simulink model "PMSM_MRAS"  (R2018b)
settings: Solver=ode23tb  StartTime=0.0  StopTime=6  FixedStep=5e-5  RelTol=1e-3  EnableMultiTasking=on
InitFcn:
  | L=8.5e-3;
  | R=2.875;
  | flux=0.175;
libraries: powerlib x5, powerlib_extras x3, simulink x1
settings Model: Creator=Paladin611  LastModifiedBy=liangjin
settings DataIOCC: SaveFormat=Array
settings OptimizationCC: ExpressionDepthLimit=2147483647  InitFltsAndDblsToZero=on  EfficientMapNaN2IntZero=off  LifeSpan=inf
settings DebuggingCC: SaveWithParameterizedLinksMsg=none  UnderspecifiedInitializationDetection=Classic  MergeDetectMultiDrivingBlocksExec=none  SignalResolutionControl=TryResolveAllWithWarning  SolverPrmCheckMsg=warning  MultiTaskDSMMsg=warning  MultiTaskCondExecSysMsg=none  FcnCallInpInsideContextMsg=warning  StateNameClashWarn=warning  SFUnexpectedBacktrackingDiag=warning  SFNoUnconditionalDefaultTransitionDiag=warning  SFExecutionAtInitializationDiag=none
settings HardwareCC: ProdBitPerPointer=32  ProdBitPerSizeT=32  ProdBitPerPtrDiffT=32  ProdLargestAtomicFloat=None  ProdIntDivRoundTo=Undefined  ProdEndianess=Unspecified  ProdWordSize=32  ProdHWDeviceType=32-bit Generic  TargetBitPerPointer=64  TargetBitPerSizeT=64  TargetBitPerPtrDiffT=64  TargetLongLongMode=on  TargetIntDivRoundTo=Zero  TargetEndianess=LittleEndian  TargetWordSize=64  TargetHWDeviceType=MATLAB Host  ProdEqTarget=off
settings ModelReferenceCC: PropagateSignalLabelsOutOfModel=off
settings SFSimCC: SimUseLocalCustomCode=off
settings RTWCC: RTWUseLocalCustomCode=off
settings CodeAppCC: MaxIdLength=128  StateflowObjectComments=on
settings GRTTargetCC: TargetLangStandard=C89/C90 (ANSI)  GeneratePreprocessorConditionals=Disable all  CombineOutputUpdateFcns=off  GRTInterface=on
settings ConfigComp: CovMetricSettings=dw  CovHtmlReporting=on  CovSaveCumulativeToWorkspaceVar=on  CovSaveSingleToWorkspaceVar=on  CovExternalEMLEnable=off  CovSFcnEnable=off
settings SimscapeCC: SimscapeNormalizeSystem=off

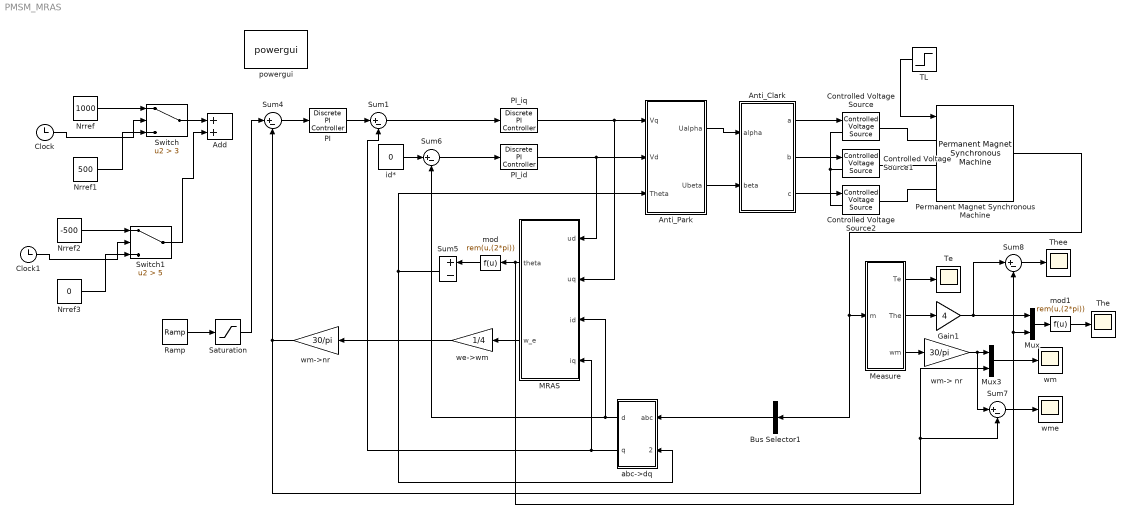
== system PMSM_MRAS ==
  Add : Sum
  Anti_Clark : Subsystem
  Anti_Park : Subsystem
  Bus Selector1 : BusSelector  OutputSignals=Stator current is_a (A),Stator current is_b (A),Stator current is_c (A)  OutputAsBus=on
  Clock : Clock
  Clock1 : Clock
  Controlled Voltage Source : powerlib/Electrical Sources/Controlled Voltage Source  Initialize=on  Source_Type=AC  Amplitude=0  Phase=0  Frequency=0  Measurements=None
      settings: SourceProductName=Simscape Electrical
  Controlled Voltage Source1 : powerlib/Electrical Sources/Controlled Voltage Source  Initialize=on  Source_Type=AC  Amplitude=0  Phase=0  Frequency=0  Measurements=None
      settings: SourceProductName=Simscape Electrical
  Controlled Voltage Source2 : powerlib/Electrical Sources/Controlled Voltage Source  Initialize=on  Source_Type=AC  Amplitude=0  Phase=0  Frequency=0  Measurements=None
      settings: SourceProductName=Simscape Electrical
  Gain1 : Gain  Gain=4
  MRAS : Subsystem
  Measure : Subsystem
  Mux : Mux  Inputs=2
  Mux3 : Mux  Inputs=2
  Nrref : Constant  Value=1000
  Nrref1 : Constant  Value=500
  Nrref2 : Constant  Value=-500
  Nrref3 : Constant  Value=0
  PI : powerlib_extras/Discrete  Control Blocks/Discrete PI Controller  Kp=0.068  Ki=17.1  Par_Limits=[60 -60]  Init=0  Ts=10e-6
  PI_id : powerlib_extras/Discrete  Control Blocks/Discrete PI Controller  Kp=L*2000  Ki=R*2000  Par_Limits=[300 -300]  Init=0  Ts=10e-6
  PI_iq : powerlib_extras/Discrete  Control Blocks/Discrete PI Controller  Kp=L*2000  Ki=R*2000  Par_Limits=[300 -300]  Init=0  Ts=10e-6
  Permanent Magnet Synchronous Machine : powerlib/Machines/Permanent Magnet Synchronous Machine  NbPhases=3  FluxDistribution=Sinusoidal  RotorType=Salient-pole  MechanicalLoad=Torque Tm  PresetModel=No  ShowDetailedParameters=on  MeasurementBus=off  Resistance=2.875  Inductance=8.5e-3  dqInductances=[8.5e-3 8.5e-3]  La=0.00085  MachineConstant=Flux linkage established by magnets (V.s)  Flux=0.175  VoltageCst=126.966  TorqueCst=1.05  Flat=120  Mechanical=[4.8e-6,0,4,0]  PolePairs=4  InitialConditions=[0,0, 0,0]  InitialConditions5ph=[0 0 0 0 0 0]  TsPowergui=0  TsBlock=-1  RefAngle=Aligned with phase A axis (original Park)
  Ramp : simulink/Sources/Ramp  slope=250  start=0  InitialOutput=0
  Saturation : Saturate  UpperLimit=1000  LowerLimit=-1000
  Sum{1,4,6..8} (5 alike) : Sum  Inputs=|+-
  Sum5 : Sum  Inputs=+-
  Switch : Switch  Criteria=u2 > Threshold  Threshold=3
  Switch1 : Switch  Criteria=u2 > Threshold  Threshold=5
  TL : Step  Time=0  SampleTime=0
  Te : Scope
  The : Scope
  Thee : Scope
  abc->dq : Subsystem
  id* : Constant  Value=0
  mod : Fcn  Expr=rem(u,(2*pi))
  mod1 : Fcn  Expr=rem(u,(2*pi))
  powergui : powerlib/powergui  Priority=1  SimulationMode=Continuous  SampleTime=1e-6  frequency=60  Iterations=50  frequencyindice=0  Pbase=100e6  ErrMax=1e-4  UnitsV=kV  UnitsW=MW  buscounter=0  FunctionMessages=off  echomessages=off  EnableUseOfTLC=off  CurrentSourceSwitches=on  DisableSnubberDevices=off  DisableRonSwitches=off  DisableVfSwitches=off  DisplayEquations=off  SolverType=Tustin  Interpol=off  ExternalGateDelay=off  methode=off  Ts=0  x0status=blocks  SPID=off  SwTol=0  HookPort=off  RestoreLinks=warning  ResistiveCurrentMeasurement=off  Frange=[0:2:500]  Ylog=off  Xlog=on  ShowGrid=off  save=off  variable=ZData  structure=0  ZoomFFT=off  StartTime=0.0  cycles=1  DisplayStyle=1  fundamental=60  FreqAxis=off  MaxFrequency=1000  frequencyindicesteady=1  RmsSteady=1  display=off
  we->wm : Gain  Gain=1/4
  wm : Scope
  wm-> nr : Gain  Gain=30/pi
  wm->nr : Gain  Gain=30/pi
  wme : Scope
  wires:
  Permanent Magnet Synchronous Machine/1 -> Bus Selector1/1, Measure/1(m)
  Sum4/1 -> PI/1
  Sum1/1 -> PI_iq/1
  Sum6/1 -> PI_id/1
  PI/1 -> Sum1/1
  ? -> Sum5/2
  id*/1 -> Sum6/1
  abc->dq/1(d) -> MRAS/3(id), Sum6/2
  abc->dq/2(q) -> Sum1/2, MRAS/4(iq)
  MRAS/2(w_e) -> we->wm/1
  we->wm/1 -> wm->nr/1
  Sum5/1 -> Anti_Park/3(Theta), abc->dq/2(theta)
  PI_iq/1 -> Anti_Park/1(Vq), MRAS/2(uq)
  PI_id/1 -> Anti_Park/2(Vd), MRAS/1(ud)
  Measure/1(Te) -> Te/1
  Measure/2(The) -> Gain1/1
  Bus Selector1/1 -> abc->dq/1(abc)
  mod/1 -> Sum5/1
  Measure/3(wm) -> wm-> nr/1
  Mux3/1 -> wm/1
  wm->nr/1 -> Sum7/2, Mux3/2, Sum4/2
  wm-> nr/1 -> Sum7/1, Mux3/1
  Sum7/1 -> wme/1
  Sum8/1 -> Thee/1
  TL/1 -> Permanent Magnet Synchronous Machine/1
  Mux/1 -> mod1/1
  Gain1/1 -> Mux/1, Sum8/1
  MRAS/1(theta) -> Sum8/2, Mux/2, mod/1
  mod1/1 -> The/1
  Anti_Park/1(Ualpha) -> Anti_Clark/1(alpha)
  Anti_Park/2(Ubeta) -> Anti_Clark/2(beta)
  Anti_Clark/1(a) -> Controlled Voltage Source/1
  Anti_Clark/2(b) -> Controlled Voltage Source1/1
  Anti_Clark/3(c) -> Controlled Voltage Source2/1
  Ramp/1 -> Saturation/1
  Nrref/1 -> Switch/1
  Nrref1/1 -> Switch/3
  Clock/1 -> Switch/2
  Switch/1 -> Add/1
  Clock1/1 -> Switch1/2
  Nrref3/1 -> Switch1/3
  Nrref2/1 -> Switch1/1
  Switch1/1 -> Add/2
  Saturation/1 -> Sum4/1
  connections:
  Controlled Voltage Source/RConn1 -- Permanent Magnet Synchronous Machine/LConn1
  Controlled Voltage Source1/RConn1 -- Permanent Magnet Synchronous Machine/LConn2
  Controlled Voltage Source2/RConn1 -- Permanent Magnet Synchronous Machine/LConn3
  Controlled Voltage Source/LConn1 -- Controlled Voltage Source2/LConn1 -- Controlled Voltage Source1/LConn1

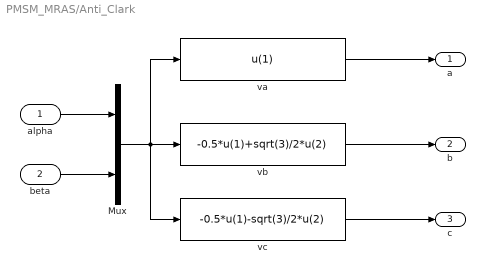
== system PMSM_MRAS/Anti_Clark ==
  alpha : Inport
  beta : Inport  Port=2
  Mux : Mux  Inputs=2
  va : Fcn  Expr=u(1)
  vb : Fcn  Expr=-0.5*u(1)+sqrt(3)/2*u(2)
  vc : Fcn  Expr=-0.5*u(1)-sqrt(3)/2*u(2)
  a : Outport
  b : Outport  Port=2
  c : Outport  Port=3
  wires:
  va/1 -> a/1
  beta/1 -> Mux/2
  alpha/1 -> Mux/1
  Mux/1 -> vc/1, vb/1, va/1
  vb/1 -> b/1
  vc/1 -> c/1

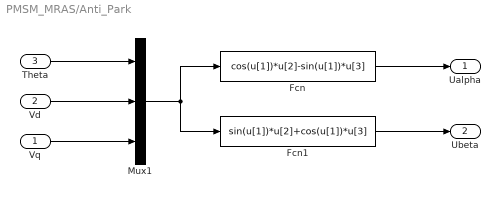
== system PMSM_MRAS/Anti_Park ==
  Vq : Inport
  Vd : Inport  Port=2
  Theta : Inport  Port=3
  Fcn : Fcn  Expr=cos(u[1])*u[2]-sin(u[1])*u[3]
  Fcn1 : Fcn  Expr=sin(u[1])*u[2]+cos(u[1])*u[3]
  Mux1 : Mux  Inputs=3
  Ualpha : Outport
  Ubeta : Outport  Port=2
  wires:
  Fcn1/1 -> Ubeta/1
  Fcn/1 -> Ualpha/1
  Mux1/1 -> Fcn/1, Fcn1/1
  Vd/1 -> Mux1/2
  Vq/1 -> Mux1/3
  Theta/1 -> Mux1/1

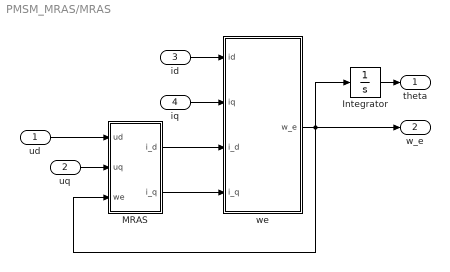
== system PMSM_MRAS/MRAS ==
  ud : Inport
  uq : Inport  Port=2
  id : Inport  Port=3
  iq : Inport  Port=4
  Integrator : Integrator
  MRAS : Subsystem
  we : Subsystem
  theta : Outport
  w_e : Outport  Port=2
  wires:
  ud/1 -> MRAS/1(ud)
  iq/1 -> we/2(iq)
  we/1(w_e) -> MRAS/3(we), w_e/1, Integrator/1
  uq/1 -> MRAS/2(uq)
  Integrator/1 -> theta/1
  MRAS/2(i_q) -> we/4(i_q)
  id/1 -> we/1(id)
  MRAS/1(i_d) -> we/3(i_d)

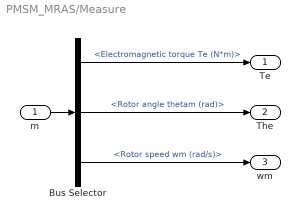
== system PMSM_MRAS/Measure ==
  m : Inport
  Bus Selector : BusSelector  OutputSignals=Electromagnetic torque Te (N*m),Rotor angle thetam (rad),Rotor speed wm (rad/s)
  Te : Outport
  The : Outport  Port=2
  wm : Outport  Port=3
  wires:
  Bus Selector/1 -> Te/1  "<Electromagnetic torque Te (N*m)>"
  Bus Selector/3 -> wm/1  "<Rotor speed wm (rad/s)>"
  Bus Selector/2 -> The/1  "<Rotor angle thetam (rad)>"
  m/1 -> Bus Selector/1

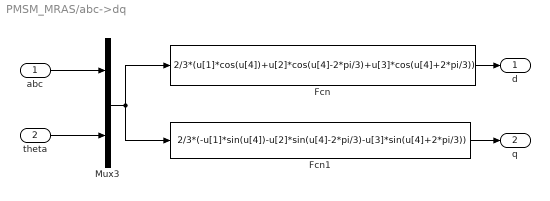
== system PMSM_MRAS/abc->dq ==
  abc : Inport
  theta : Inport  Port=2
  Fcn : Fcn  Expr=2/3*(u[1]*cos(u[4])+u[2]*cos(u[4]-2*pi/3)+u[3]*cos(u[4]+2*pi/3))
  Fcn1 : Fcn  Expr=2/3*(-u[1]*sin(u[4])-u[2]*sin(u[4]-2*pi/3)-u[3]*sin(u[4]+2*pi/3))
  Mux3 : Mux  Inputs=2
  d : Outport
  q : Outport  Port=2
  wires:
  Mux3/1 -> Fcn1/1, Fcn/1
  theta/1 -> Mux3/2
  Fcn/1 -> d/1
  Fcn1/1 -> q/1
  abc/1 -> Mux3/1

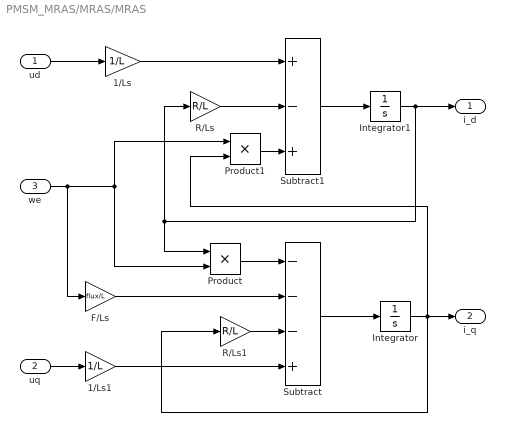
== system PMSM_MRAS/MRAS/MRAS ==
  ud : Inport
  uq : Inport  Port=2
  we : Inport  Port=3
  1/Ls : Gain  Gain=1/L
  1/Ls1 : Gain  Gain=1/L
  F/Ls : Gain  Gain=flux/L
  Integrator : Integrator
  Integrator1 : Integrator
  Product : Product  RndMeth=Zero
  Product1 : Product  RndMeth=Zero
  R/Ls : Gain  Gain=R/L
  R/Ls1 : Gain  Gain=R/L
  Subtract : Sum  Inputs=---+
  Subtract1 : Sum  Inputs=+-+
  i_d : Outport
  i_q : Outport  Port=2
  wires:
  1/Ls1/1 -> Subtract/4
  Subtract/1 -> Integrator/1
  Subtract1/1 -> Integrator1/1
  1/Ls/1 -> Subtract1/1
  Product1/1 -> Subtract1/3
  R/Ls/1 -> Subtract1/2
  Product/1 -> Subtract/1
  R/Ls1/1 -> Subtract/3
  uq/1 -> 1/Ls1/1
  we/1 -> F/Ls/1, Product/2, Product1/1
  F/Ls/1 -> Subtract/2
  Integrator1/1 -> R/Ls/1, Product/1, i_d/1
  ud/1 -> 1/Ls/1
  Integrator/1 -> R/Ls1/1, i_q/1, Product1/2

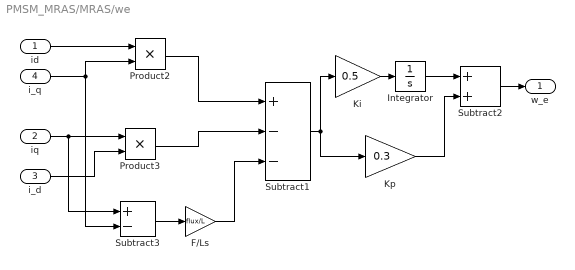
== system PMSM_MRAS/MRAS/we ==
  id : Inport
  iq : Inport  Port=2
  i_d : Inport  Port=3
  i_q : Inport  Port=4
  F/Ls : Gain  Gain=flux/L
  Integrator : Integrator
  Ki : Gain  Gain=0.5
  Kp : Gain  Gain=0.3
  Product2 : Product  RndMeth=Zero
  Product3 : Product  RndMeth=Zero
  Subtract1 : Sum  Inputs=+--
  Subtract2 : Sum
  Subtract3 : Sum  Inputs=+-
  w_e : Outport
  wires:
  id/1 -> Product2/1
  i_q/1 -> Subtract3/2, Product2/2
  iq/1 -> Subtract3/1, Product3/1
  i_d/1 -> Product3/2
  Subtract3/1 -> F/Ls/1
  F/Ls/1 -> Subtract1/3
  Subtract1/1 -> Ki/1, Kp/1
  Ki/1 -> Integrator/1
  Integrator/1 -> Subtract2/1
  Kp/1 -> Subtract2/2
  Product2/1 -> Subtract1/1
  Product3/1 -> Subtract1/2
  Subtract2/1 -> w_e/1
